simulink model "funkcia21"  (R2020a)
settings: Solver=VariableStepAuto  StartTime=0.0  StopTime=10.0  RelTol=1e-3
libraries: simulink x1
settings Model: Creator=xacha  LastModifiedBy=xacha

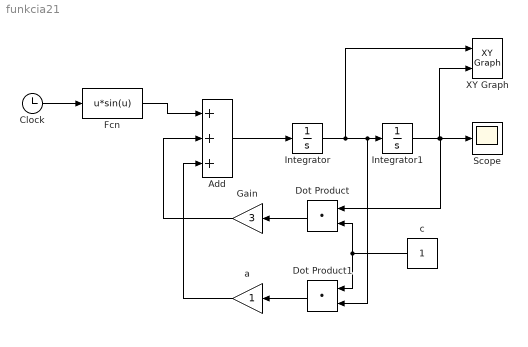
== system funkcia21 ==
  Add : Sum  Inputs=+++
  Clock : Clock
  Dot Product : DotProduct  InputSameDT=on  OutDataTypeStr=Inherit: Inherit via internal rule
  Dot Product1 : DotProduct  InputSameDT=on  OutDataTypeStr=Inherit: Inherit via internal rule
  Fcn : Fcn  Expr=u*sin(u)
  Gain : Gain  Gain=3  mask{constant3=0}
      mask prompts: constant3 "constant 3"
  Integrator : Integrator
  Integrator1 : Integrator
  Scope : Scope
  XY Graph : simulink/Sinks/XY Graph  xmin=-1  xmax=1  ymin=-1  ymax=1  st=-1
  a : Gain  mask{a=0}
      mask prompts: a "input a"
  c : Constant  mask{c=0}
      mask prompts: c "input c"
  wires:
  Dot Product/1 -> Gain/1
  Gain/1 -> Add/2
  a/1 -> Add/3
  Dot Product1/1 -> a/1
  c/1 -> Dot Product1/1, Dot Product/2
  Integrator1/1 -> XY Graph/2, Dot Product/1, Scope/1
  Integrator/1 -> Integrator1/1, Dot Product1/2, XY Graph/1
  Fcn/1 -> Add/1
  Add/1 -> Integrator/1
  Clock/1 -> Fcn/1
